simulink model "Root_Locus_Controller"  (R2024a)
settings: Solver=VariableStepAuto  StartTime=0.0  StopTime=100  RelTol=1e-3
libraries: simulink x1
settings Model: Creator=tinas  LastModifiedBy=LENOVO

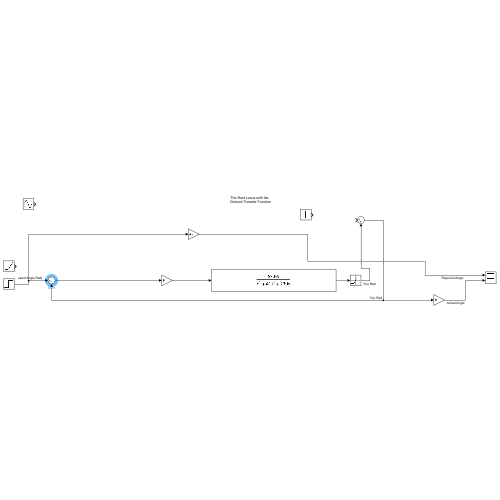
[thumbnail: Simulink's stored preview of the top-level diagram]
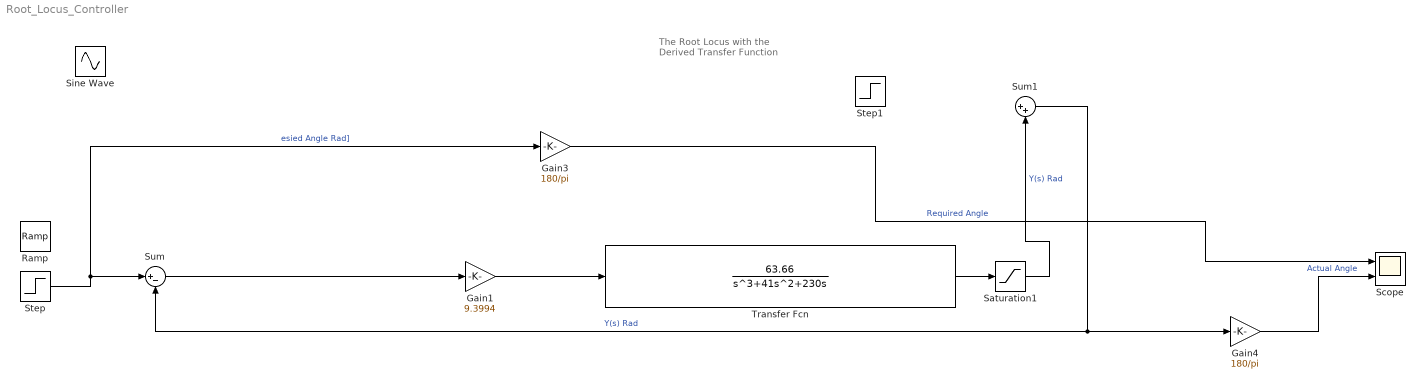
== system Root_Locus_Controller ==
  note: The Root Locus with the Derived Transfer Function
  Gain1 : Gain  Gain=9.3994
  Gain3 : Gain  Gain=180/pi
  Gain4 : Gain  Gain=180/pi
  Ramp : simulink/Sources/Ramp  slope=(120*pi/180)/(12*3600)  start=0  InitialOutput=0
  Saturation1 : Saturate  UpperLimit=135*pi/180  LowerLimit=-pi/2
  Scope : Scope  NumInputPorts=2
  Sine Wave : Sin  Amplitude=10*pi/180  SampleTime=0
  Step : Step  Time=0  After=45*pi/180  SampleTime=0
  Step1 : Step  Time=10  After=15*pi/180  SampleTime=0
  Sum : Sum  Inputs=|+-
  Sum1 : Sum  Inputs=|++
  Transfer Fcn : TransferFcn  Numerator=[63.66]  Denominator="[1   41  230  0]"
  wires:
  Gain1/1 -> Transfer Fcn/1
  Step/1 -> Gain3/1, Sum/1  "esied Angle Rad]"
  Transfer Fcn/1 -> Saturation1/1
  Sum1/1 -> Gain4/1, Sum/2  "Y(s) Rad"
  Gain3/1 -> Scope/1  "Required Angle"
  Gain4/1 -> Scope/2  "Actual Angle"
  Saturation1/1 -> Sum1/2  "Y(s) Rad"
  Sum/1 -> Gain1/1
